simulink model "blocks"  (Simulink 3.00)
settings: Solver=ode45  SolverMode=SingleTasking  StartTime=0.0  StopTime=10.0  RelTol=1e-3  AbsTol=1e-6
undefined symbols (not defined in the file): C, L, R
settings Model: LastModifiedBy=eechris

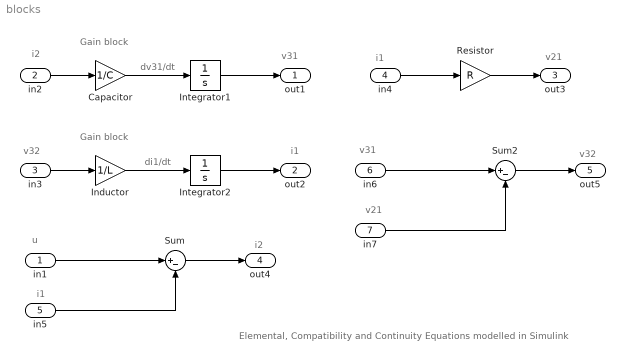
== system blocks ==
  note: dv31/dt
  note: v31
  note: Gain block
  note: di1/dt
  note: i1
  note: Gain block
  note: i2
  note: i1
  note: v21
  note: v32
  note: u
  note: i1
  note: i2
  note: v31
  note: v21
  note: v32
  note: Elemental, Compatibility and Continuity Equations modelled in Simulink
  in1 : Inport  Port=1  PortWidth=-1  SampleTime=-1  DataType=auto
      settings: SignalType=auto
  in2 : Inport  Port=2  PortWidth=-1  SampleTime=-1  DataType=auto
      settings: SignalType=auto
  in3 : Inport  Port=3  PortWidth=-1  SampleTime=-1  DataType=auto
      settings: SignalType=auto
  in4 : Inport  Port=4  PortWidth=-1  SampleTime=-1  DataType=auto
      settings: SignalType=auto
  in5 : Inport  Port=5  PortWidth=-1  SampleTime=-1  DataType=auto
      settings: SignalType=auto
  in6 : Inport  Port=6  PortWidth=-1  SampleTime=-1  DataType=auto
      settings: SignalType=auto
  in7 : Inport  Port=7  PortWidth=-1  SampleTime=-1  DataType=auto
      settings: SignalType=auto
  Capacitor : Gain  Gain=1/C  SaturateOnIntegerOverflow=off
  Inductor : Gain  Gain=1/L  SaturateOnIntegerOverflow=off
  Integrator1 : Integrator  ExternalReset=none  InitialConditionSource=internal  InitialCondition=0  LimitOutput=off  UpperSaturationLimit=inf  LowerSaturationLimit=-inf  ShowSaturationPort=off  ShowStatePort=off  AbsoluteTolerance=auto
  Integrator2 : Integrator  ExternalReset=none  InitialConditionSource=internal  InitialCondition=0  LimitOutput=off  UpperSaturationLimit=inf  LowerSaturationLimit=-inf  ShowSaturationPort=off  ShowStatePort=off  AbsoluteTolerance=auto
  Resistor : Gain  Gain=R  SaturateOnIntegerOverflow=on
  Sum : Sum  Inputs=|+-  SaturateOnIntegerOverflow=off
  Sum2 : Sum  Inputs=|+-  SaturateOnIntegerOverflow=off
  out1 : Outport  Port=1
  out2 : Outport  Port=2
  out3 : Outport  Port=3
  out4 : Outport  Port=4
  out5 : Outport  Port=5
  wires:
  Capacitor/1 -> Integrator1/1
  in2/1 -> Capacitor/1
  Integrator1/1 -> out1/1
  Inductor/1 -> Integrator2/1
  in3/1 -> Inductor/1
  Integrator2/1 -> out2/1
  in4/1 -> Resistor/1
  Resistor/1 -> out3/1
  in6/1 -> Sum2/1
  Sum2/1 -> out5/1
  in7/1 -> Sum2/2
  in1/1 -> Sum/1
  Sum/1 -> out4/1
  in5/1 -> Sum/2
